simulink model "MR_SOC_SOP_SOE_Estimator"  (R2022b)
settings: Solver=VariableStepAuto  StartTime=0.0  StopTime=10.0  RelTol=1e-3
undefined symbols (not defined in the file): Initial_Covariance, L_SOP, MaxChargeCurrent, MaxDischargeCurrent, Measurement_Noise_Covariance, NumberSt, NumModules, NumParallel, NumSeries, OCV_25, Process_Noise_Covariance, SOC_Max, SOC_Min, SOC_Vec1, SOH_Vec, Temperature_Vec, Ts, Ts_SOP, Vmax, Vmin
settings Model: DataDictionary=Estimators_Dictionary.sldd  Creator=japerez  LastModifiedBy=jgavidia
settings DebuggingCC: ParameterPrecisionLossMsg=none

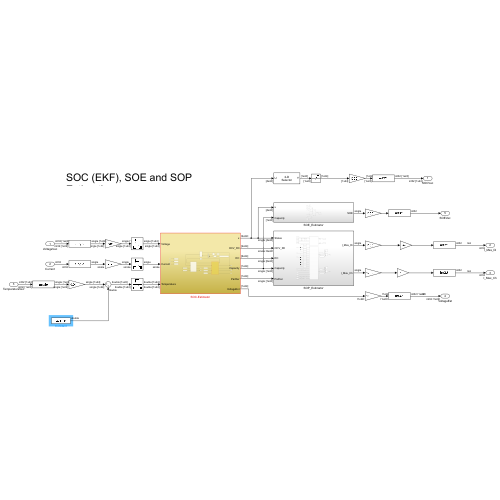
[thumbnail: Simulink's stored preview of the top-level diagram]
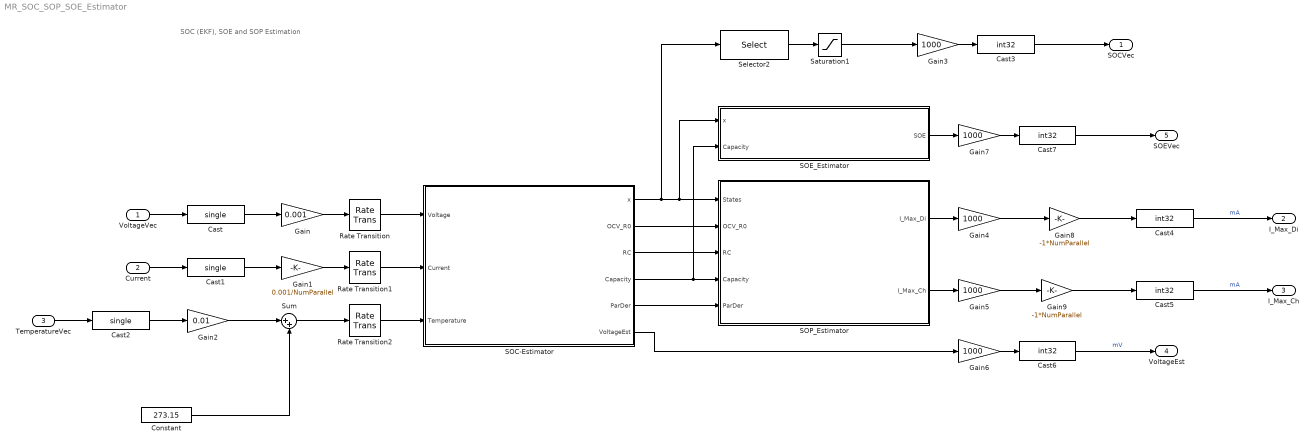
== system MR_SOC_SOP_SOE_Estimator ==
  note: SOC (EKF), SOE and SOP Estimation
  VoltageVec : Inport  OutDataTypeStr=int32  PortDimensions=[1,NumSeries*NumModules]
  Current : Inport  Port=2  OutDataTypeStr=int32  PortDimensions=1
  TemperatureVec : Inport  Port=3  OutDataTypeStr=int32  PortDimensions=[1,NumSeries*NumModules]
  Cast : DataTypeConversion  OutDataTypeStr=single  SaturateOnIntegerOverflow=off  RndMeth=Floor
  Cast1 : DataTypeConversion  OutDataTypeStr=single  SaturateOnIntegerOverflow=off  RndMeth=Floor
  Cast2 : DataTypeConversion  OutDataTypeStr=single  SaturateOnIntegerOverflow=off  RndMeth=Floor
  Cast{3..7} (5 alike) : DataTypeConversion  OutDataTypeStr=int32  SaturateOnIntegerOverflow=off  RndMeth=Floor
  Constant : Constant  Value=273.15  OutDataTypeStr=single
  Gain : Gain  Gain=0.001
  Gain1 : Gain  Gain=0.001/NumParallel
  Gain2 : Gain  Gain=0.01
  Gain{3..7} (5 alike) : Gain  Gain=1000
  Gain8 : Gain  Gain=-1*NumParallel
  Gain9 : Gain  Gain=-1*NumParallel
  Rate Transition : RateTransition  Integrity=off  OutPortSampleTime=Ts
  Rate Transition1 : RateTransition  Integrity=off  OutPortSampleTime=Ts
  Rate Transition2 : RateTransition  Integrity=off  OutPortSampleTime=Ts
  SOC-Estimator : Subsystem
  SOE_Estimator : Subsystem
  SOP_Estimator : Subsystem
  Saturation1 : Saturate  UpperLimit=1  LowerLimit=0
  Selector2 : Selector  NumberOfDimensions=2  InputPortWidth=24  IndexOptions=Index vector (dialog),Select all  Indices=1,1  OutputSizes=1,1
  Sum : Sum  Inputs=|++
  SOCVec : Outport  OutDataTypeStr=int32  PortDimensions=[1,NumSeries*NumModules]
  I_Max_Di : Outport  Port=2  OutDataTypeStr=int32  PortDimensions=1
  I_Max_Ch : Outport  Port=3  OutDataTypeStr=int32  PortDimensions=1
  VoltageEst : Outport  Port=4  OutDataTypeStr=int32  PortDimensions=[1,NumSeries*NumModules]
  SOEVec : Outport  Port=5
  wires:
  Gain/1 -> Rate Transition/1
  Rate Transition2/1 -> SOC-Estimator/3(Temperature)
  Gain1/1 -> Rate Transition1/1
  Selector2/1 -> Saturation1/1
  VoltageVec/1 -> Cast/1
  Current/1 -> Cast1/1
  TemperatureVec/1 -> Cast2/1
  Cast/1 -> Gain/1
  Cast1/1 -> Gain1/1
  Cast2/1 -> Gain2/1
  Gain3/1 -> Cast3/1
  Saturation1/1 -> Gain3/1
  SOC-Estimator/1(x) -> SOE_Estimator/1(x), SOP_Estimator/1(States), Selector2/1
  SOC-Estimator/2(OCV_R0) -> SOP_Estimator/2(OCV_R0)
  SOC-Estimator/3(RC) -> SOP_Estimator/3(RC)
  SOC-Estimator/4(Capacity) -> SOE_Estimator/2(Capacity), SOP_Estimator/4(Capacity)
  SOC-Estimator/5(ParDer) -> SOP_Estimator/5(ParDer)
  SOP_Estimator/1(I_Max_Di) -> Gain4/1
  SOP_Estimator/2(I_Max_Ch) -> Gain5/1
  Gain6/1 -> Cast6/1
  SOC-Estimator/6(VoltageEst) -> Gain6/1
  Rate Transition1/1 -> SOC-Estimator/2(Current)
  Rate Transition/1 -> SOC-Estimator/1(Voltage)
  Cast3/1 -> SOCVec/1
  Cast4/1 -> I_Max_Di/1  "mA"
  Cast5/1 -> I_Max_Ch/1  "mA"
  Cast6/1 -> VoltageEst/1  "mV"
  SOE_Estimator/1(SOE) -> Gain7/1
  Gain7/1 -> Cast7/1
  Cast7/1 -> SOEVec/1
  Constant/1 -> Sum/2
  Gain2/1 -> Sum/1
  Sum/1 -> Rate Transition2/1
  Gain5/1 -> Gain9/1
  Gain9/1 -> Cast5/1
  Gain4/1 -> Gain8/1
  Gain8/1 -> Cast4/1

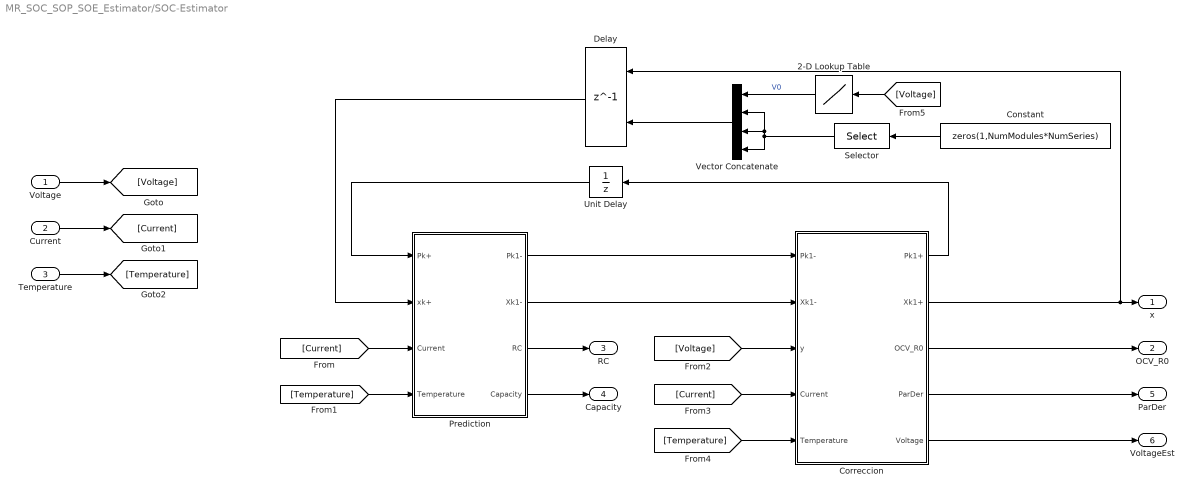
== system MR_SOC_SOP_SOE_Estimator/SOC-Estimator ==
  Voltage : Inport
  Current : Inport  Port=2
  Temperature : Inport  Port=3
  2-D Lookup Table : Lookup_n-D  NumberOfTableDimensions=1  BreakpointsForDimension1=OCV_25  BreakpointsForDimension2=Temperature_Vec  BreakpointsForDimension3=SOH_Vec  Table=SOC_Vec1  ExtrapMethod=Clip  InternalRulePriority=Speed  RndMeth=Simplest
  Constant : Constant  Value=zeros(1,NumModules*NumSeries)  OutDataTypeStr=single
  Correccion : Subsystem
  Delay : Delay  DelayLength=1  InitialConditionSource=Input port
      settings: InputPortMap=u0,p4
  Prediction : Subsystem
  Selector : Selector  NumberOfDimensions=2  InputPortWidth=3  IndexOptions=Select all,Index vector (dialog)  Indices=[1 3],[1:24]  OutputSizes=1,1
  Unit Delay : UnitDelay  InitialCondition=Initial_Covariance.*ones(NumberSt, NumModules*NumSeries)  SampleTime=Ts  HasFrameUpgradeWarning=on
  Vector Concatenate : Concatenate  NumInputs=4  Mode=Multidimensional array
  x : Outport
  OCV_R0 : Outport  Port=2
  RC : Outport  Port=3
  Capacity : Outport  Port=4
  ParDer : Outport  Port=5
  VoltageEst : Outport  Port=6
  wires:
  [Current] -> Prediction/3(Current)
  [Temperature] -> Prediction/4(Temperature)
  Temperature/1 -> [Temperature]
  Correccion/1(Pk1+) -> Unit Delay/1
  Prediction/1(Pk1-) -> Correccion/1(Pk1-)
  Prediction/2(Xk1-) -> Correccion/2(Xk1-)
  Correccion/2(Xk1+) -> Delay/1, x/1
  [Voltage] -> Correccion/3(y)
  Voltage/1 -> [Voltage]
  Current/1 -> [Current]
  Unit Delay/1 -> Prediction/1(Pk+)
  [Temperature] -> Correccion/5(Temperature)
  [Current] -> Correccion/4(Current)
  Correccion/3(OCV_R0) -> OCV_R0/1
  Delay/1 -> Prediction/2(xk+)
  Prediction/3(RC) -> RC/1
  Prediction/4(Capacity) -> Capacity/1
  Correccion/4(ParDer) -> ParDer/1
  Correccion/5(Voltage) -> VoltageEst/1
  Constant/1 -> Selector/1
  2-D Lookup Table/1 -> Vector Concatenate/1  "V0"
  Vector Concatenate/1 -> Delay/2
  [Voltage] -> 2-D Lookup Table/1
  Selector/1 -> Vector Concatenate/2, Vector Concatenate/3, Vector Concatenate/4

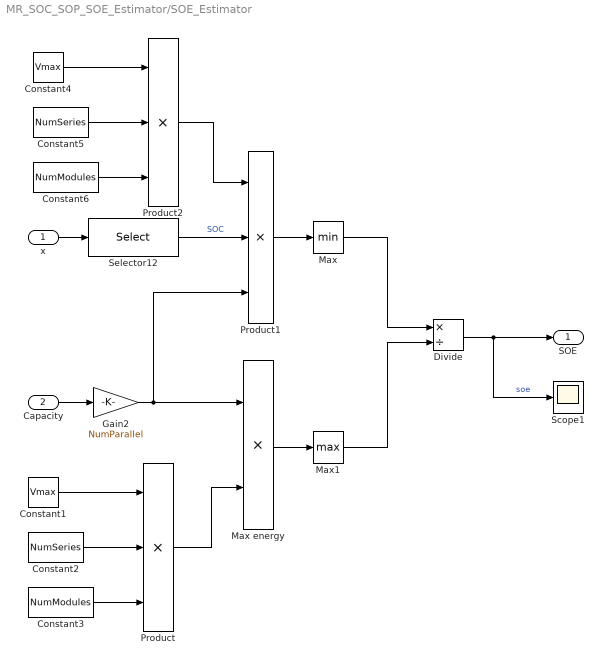
== system MR_SOC_SOP_SOE_Estimator/SOE_Estimator ==
  x : Inport
  Capacity : Inport  Port=2
  Constant1 : Constant  Value=Vmax
  Constant2 : Constant  Value=NumSeries
  Constant3 : Constant  Value=NumModules
  Constant4 : Constant  Value=Vmax
  Constant5 : Constant  Value=NumSeries
  Constant6 : Constant  Value=NumModules
  Divide : Product  Inputs=*/
  Gain2 : Gain  Gain=NumParallel
  Max : MinMax
  Max energy : Product
  Max1 : MinMax  Function=max
  Product : Product  Inputs=3
  Product1 : Product  Inputs=3
  Product2 : Product  Inputs=3
  Scope1 : Scope
  Selector12 : Selector  NumberOfDimensions=2  InputPortWidth=24  IndexOptions=Index vector (dialog),Select all  Indices=1,1  OutputSizes=1,1
  SOE : Outport  OutDataTypeStr=single
  wires:
  x/1 -> Selector12/1
  Constant1/1 -> Product/1
  Constant2/1 -> Product/2
  Capacity/1 -> Gain2/1
  Product/1 -> Max energy/2
  Max/1 -> Divide/1
  Max1/1 -> Divide/2
  Divide/1 -> SOE/1, Scope1/1  "soe"
  Product1/1 -> Max/1
  Max energy/1 -> Max1/1
  Constant3/1 -> Product/3
  Selector12/1 -> Product1/2  "SOC"
  Constant6/1 -> Product2/3
  Constant5/1 -> Product2/2
  Constant4/1 -> Product2/1
  Product2/1 -> Product1/1
  Gain2/1 -> Product1/3, Max energy/1

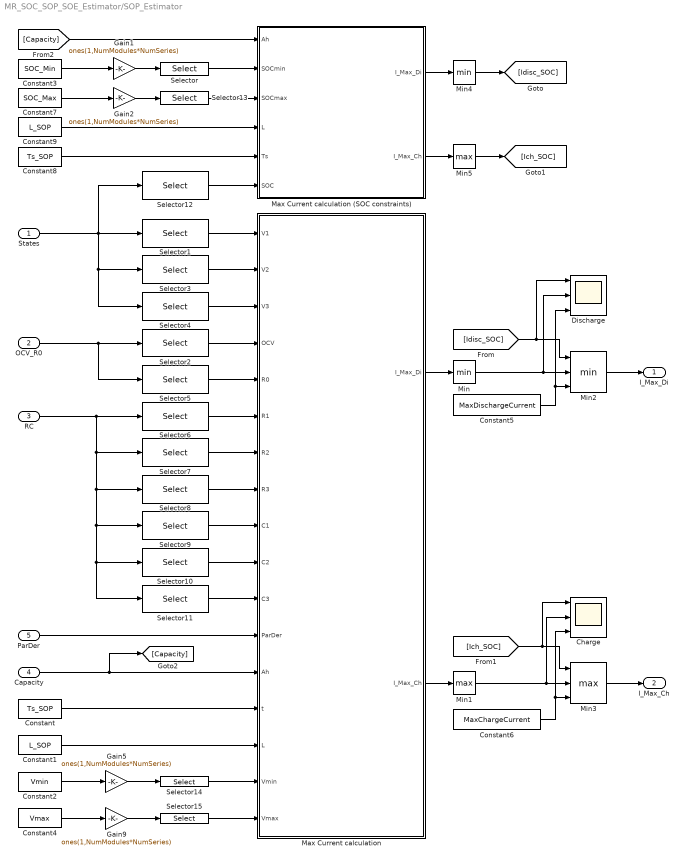
== system MR_SOC_SOP_SOE_Estimator/SOP_Estimator ==
  States : Inport  OutDataTypeStr=single  PortDimensions=[NumberSt, NumModules*NumSeries]
  OCV_R0 : Inport  Port=2  OutDataTypeStr=single  PortDimensions=[2,NumModules*NumSeries]
  RC : Inport  Port=3  OutDataTypeStr=single  PortDimensions=[6,NumModules*NumSeries]
  Capacity : Inport  Port=4  OutDataTypeStr=single  PortDimensions=[1,NumModules*NumSeries]
  ParDer : Inport  Port=5  OutDataTypeStr=single  PortDimensions=[1,NumModules*NumSeries]
  Charge : Scope  NumInputPorts=3
  Constant : Constant  Value=Ts_SOP
  Constant1 : Constant  Value=L_SOP
  Constant2 : Constant  Value=Vmin  OutDataTypeStr=single
  Constant3 : Constant  Value=SOC_Min  OutDataTypeStr=single
  Constant4 : Constant  Value=Vmax  OutDataTypeStr=single
  Constant5 : Constant  Value=MaxDischargeCurrent
  Constant6 : Constant  Value=MaxChargeCurrent
  Constant7 : Constant  Value=SOC_Max  OutDataTypeStr=single
  Constant8 : Constant  Value=Ts_SOP
  Constant9 : Constant  Value=L_SOP
  Discharge : Scope  NumInputPorts=3
  Gain{1..2,5,9} (4 alike) : Gain  Gain=ones(1,NumModules*NumSeries)  ParamDataTypeStr=single  OutDataTypeStr=single
  Max Current calculation : MATLAB Function  TreatAsAtomicUnit=on
  Max Current calculation (SOC constraints) : MATLAB Function  TreatAsAtomicUnit=on
  Min : MinMax
  Min1 : MinMax  Function=max
  Min2 : MinMax  Inputs=3
  Min3 : MinMax  Function=max  Inputs=3
  Min4 : MinMax
  Min5 : MinMax  Function=max
  Selector{,13..15} (4 alike) : Selector  NumberOfDimensions=2  InputPortWidth=3  IndexOptions=Index vector (dialog),Select all  Indices=1,1  OutputSizes=1,1
  Selector1 : Selector  NumberOfDimensions=2  InputPortWidth=24  IndexOptions=Index vector (dialog),Select all  Indices=2,2  OutputSizes=1,1
  Selector10 : Selector  NumberOfDimensions=2  InputPortWidth=24  IndexOptions=Index vector (dialog),Select all  Indices=5,5  OutputSizes=1,1
  Selector11 : Selector  NumberOfDimensions=2  InputPortWidth=24  IndexOptions=Index vector (dialog),Select all  Indices=6,6  OutputSizes=1,1
  Selector12 : Selector  NumberOfDimensions=2  InputPortWidth=24  IndexOptions=Index vector (dialog),Select all  Indices=1,1  OutputSizes=1,1
  Selector2 : Selector  NumberOfDimensions=2  InputPortWidth=24  IndexOptions=Index vector (dialog),Select all  Indices=1,1  OutputSizes=1,1
  Selector3 : Selector  NumberOfDimensions=2  InputPortWidth=24  IndexOptions=Index vector (dialog),Select all  Indices=3,3  OutputSizes=1,1
  Selector4 : Selector  NumberOfDimensions=2  InputPortWidth=24  IndexOptions=Index vector (dialog),Select all  Indices=4,4  OutputSizes=1,1
  Selector5 : Selector  NumberOfDimensions=2  InputPortWidth=24  IndexOptions=Index vector (dialog),Select all  Indices=2,2  OutputSizes=1,1
  Selector6 : Selector  NumberOfDimensions=2  InputPortWidth=24  IndexOptions=Index vector (dialog),Select all  Indices=1,1  OutputSizes=1,1
  Selector7 : Selector  NumberOfDimensions=2  InputPortWidth=24  IndexOptions=Index vector (dialog),Select all  Indices=2,2  OutputSizes=1,1
  Selector8 : Selector  NumberOfDimensions=2  InputPortWidth=24  IndexOptions=Index vector (dialog),Select all  Indices=3,3  OutputSizes=1,1
  Selector9 : Selector  NumberOfDimensions=2  InputPortWidth=24  IndexOptions=Index vector (dialog),Select all  Indices=4,4  OutputSizes=1,1
  I_Max_Di : Outport  OutDataTypeStr=single  PortDimensions=1
  I_Max_Ch : Outport  Port=2  OutDataTypeStr=single  PortDimensions=1
  wires:
  Selector1/1 -> Max Current calculation/1(V1)
  Selector5/1 -> Max Current calculation/5(R0)
  Constant2/1 -> Gain5/1
  Max Current calculation/2(I_Max_Ch) -> Min1/1
  Min2/1 -> I_Max_Di/1
  Max Current calculation/1(I_Max_Di) -> Min/1
  Constant4/1 -> Gain9/1
  OCV_R0/1 -> Selector5/1, Selector2/1
  Gain5/1 -> Selector14/1
  Capacity/1 -> [Capacity], Max Current calculation/13(Ah)
  Selector3/1 -> Max Current calculation/2(V2)
  Min3/1 -> I_Max_Ch/1
  RC/1 -> Selector11/1, Selector10/1, Selector9/1, Selector8/1, Selector7/1, Selector6/1
  Selector2/1 -> Max Current calculation/4(OCV)
  Selector6/1 -> Max Current calculation/6(R1)
  Selector11/1 -> Max Current calculation/11(C3)
  Selector10/1 -> Max Current calculation/10(C2)
  Selector9/1 -> Max Current calculation/9(C1)
  ParDer/1 -> Max Current calculation/12(ParDer)
  Selector8/1 -> Max Current calculation/8(R3)
  Selector7/1 -> Max Current calculation/7(R2)
  Selector4/1 -> Max Current calculation/3(V3)
  Constant1/1 -> Max Current calculation/15(L)
  Gain9/1 -> Selector15/1
  Constant3/1 -> Gain1/1
  States/1 -> Selector12/1, Selector4/1, Selector3/1, Selector1/1
  Constant7/1 -> Gain2/1
  Selector12/1 -> Max Current calculation (SOC constraints)/6(SOC)
  Gain2/1 -> Selector13/1
  Gain1/1 -> Selector/1
  Max Current calculation (SOC constraints)/1(I_Max_Di) -> Min4/1
  Max Current calculation (SOC constraints)/2(I_Max_Ch) -> Min5/1
  Min4/1 -> [Idisc_SOC]
  Min5/1 -> [Ich_SOC]
  Min/1 -> Discharge/2, Min2/2
  [Idisc_SOC] -> Discharge/1, Min2/1
  Constant6/1 -> Min3/3, Charge/3
  [Ich_SOC] -> Charge/1, Min3/1
  [Capacity] -> Max Current calculation (SOC constraints)/1(Ah)
  Min1/1 -> Charge/2, Min3/2
  Constant5/1 -> Discharge/3, Min2/3
  Constant9/1 -> Max Current calculation (SOC constraints)/4(L)
  Constant8/1 -> Max Current calculation (SOC constraints)/5(Ts)
  Constant/1 -> Max Current calculation/14(t)
  Selector/1 -> Max Current calculation (SOC constraints)/2(SOCmin)
  Selector13/1 -> Max Current calculation (SOC constraints)/3(SOCmax)
  Selector14/1 -> Max Current calculation/16(Vmin)
  Selector15/1 -> Max Current calculation/17(Vmax)

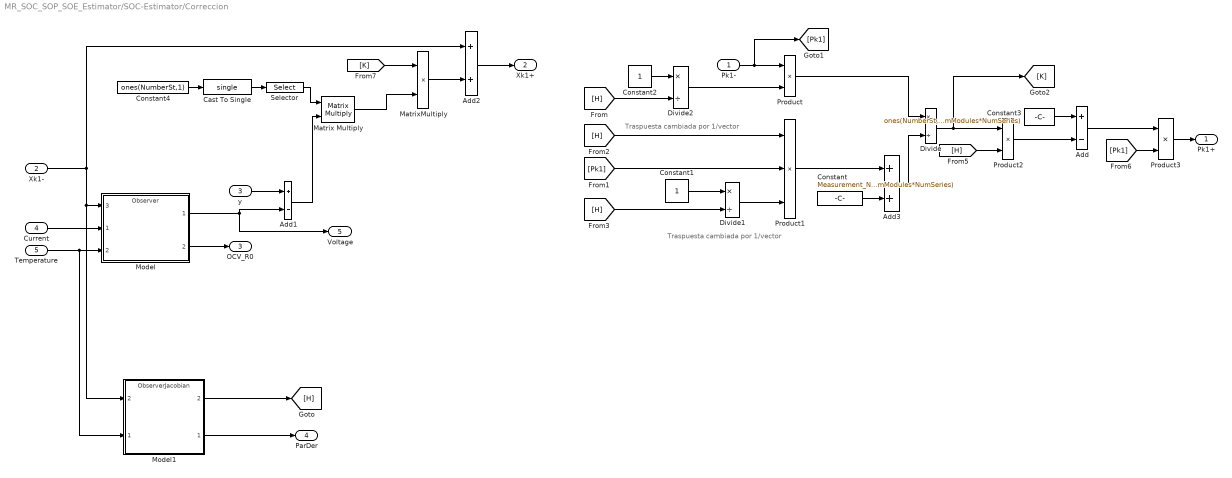
== system MR_SOC_SOP_SOE_Estimator/SOC-Estimator/Correccion ==
  note: Traspuesta cambiada por 1/vector
  note: Traspuesta cambiada por 1/vector
  Pk1- : Inport
  Xk1- : Inport  Port=2
  y : Inport  Port=3
  Current : Inport  Port=4
  Temperature : Inport  Port=5
  Add : Sum  Inputs=+-
  Add1 : Sum  Inputs=+-
  Add2 : Sum
  Add3 : Sum
  Cast To Single : DataTypeConversion  OutDataTypeStr=single  SaturateOnIntegerOverflow=off  RndMeth=Floor
  Constant : Constant  Value=Measurement_Noise_Covariance.*ones(1,NumModules*NumSeries)
  Constant1 : Constant  OutDataTypeStr=single
  Constant2 : Constant  OutDataTypeStr=single
  Constant3 : Constant  Value=ones(NumberSt,NumModules*NumSeries)  OutDataTypeStr=single
  Constant4 : Constant  Value=ones(NumberSt,1)
  Divide : Product  Inputs=*/
  Divide1 : Product  Inputs=*/
  Divide2 : Product  Inputs=*/
  Matrix Multiply : Product  Multiplication=Matrix(*)
  MatrixMultiply : Product
  Model : ModelReference  ModelNameDialog=Observer.slx  SimulationMode=Normal  ModelReferenceVersion=1.68
      settings: PortSchema="{\"entries\":[{\"content\":{\"sides\":[{\"content\":{\"connectorIds\":[\"In3\",\"In1\",\"In2\"]},\"type\":\"ConnectorPlacement.EquallySpacedRectSide\",\"uuid\":\"578ab670-1fda-43cf-957f-d385bd038916\"},{\"content\":{\"connectorIds\":[\"Out1\",\"Out2\"],\"side\":\"RIGHT\"},\"type\":\"ConnectorPlacement.EquallySpacedRectSide\",\"uuid\":\"4b969430-feda-42b7-9c79-ebef60756efb\"},{\"content\":{\"connectorIds\":[],\"side\":\"TOP\"},\"type\":\"ConnectorPlacement.EquallySpacedRectSide\",\"uuid\":\"4cac5d2b-0234-4ed0-b02b-747a59c7157b\"}]},\"type\":\"ConnectorPlacement.EquallySpacedConnector\",\"uuid\":\"85d93a1c-d19f-40da-bbe5-909812e617d2\"}],\"packageUris\":[\"http://schema.mathworks.com/mf0/Connector/R2020b\"],\"version\":\"1.0\"}"
  Model1 : ModelReference  ModelNameDialog=ObserverJacobian.slx  SimulationMode=Normal  ModelReferenceVersion=1.67
      settings: PortSchema="{\"entries\":[{\"content\":{\"sides\":[{\"content\":{\"connectorIds\":[\"In2\",\"In1\"]},\"type\":\"ConnectorPlacement.EquallySpacedRectSide\",\"uuid\":\"624b1806-31b3-4d4e-aaed-5849830d0be2\"},{\"content\":{\"connectorIds\":[\"Out2\",\"Out1\"],\"side\":\"RIGHT\"},\"type\":\"ConnectorPlacement.EquallySpacedRectSide\",\"uuid\":\"bbfd7499-df97-4924-a8a8-c1065b8018b2\"},{\"content\":{\"connectorIds\":[],\"side\":\"TOP\"},\"type\":\"ConnectorPlacement.EquallySpacedRectSide\",\"uuid\":\"a9ee114e-551d-4138-9f4b-27e93fc3876b\"}]},\"type\":\"ConnectorPlacement.EquallySpacedConnector\",\"uuid\":\"be93e1de-0c8b-49c5-8782-6d924248437e\"}],\"packageUris\":[\"http://schema.mathworks.com/mf0/Connector/R2020b\"],\"version\":\"1.0\"}"
  Product : Product
  Product1 : Product  Inputs=3
  Product2 : Product
  Product3 : Product
  Selector : Selector  NumberOfDimensions=2  InputPortWidth=3  IndexOptions=Index vector (dialog),Select all  Indices=[1 2 3 4],1  OutputSizes=1,1
  Pk1+ : Outport
  Xk1+ : Outport  Port=2
  OCV_R0 : Outport  Port=3
  ParDer : Outport  Port=4
  Voltage : Outport  Port=5
  wires:
  Pk1-/1 -> [Pk1], Product/1
  Model1/2 -> [H]
  Divide2/1 -> Product/2
  Product/1 -> Divide/1
  [H] -> Product1/1
  [Pk1] -> Product1/2
  Divide1/1 -> Product1/3
  Product1/1 -> Add3/1
  Product2/1 -> Add/2
  [H] -> Product2/2
  Add/1 -> Product3/1
  [Pk1] -> Product3/2
  Product3/1 -> Pk1+/1
  y/1 -> Add1/1
  Model/1 -> Add1/2, Voltage/1
  MatrixMultiply/1 -> Add2/2
  Xk1-/1 -> Model1/2, Model/3, Add2/1
  Add2/1 -> Xk1+/1
  Add3/1 -> Divide/2
  Current/1 -> Model/1
  Temperature/1 -> Model1/1, Model/2
  Constant1/1 -> Divide1/1
  [H] -> Divide1/2
  [H] -> Divide2/2
  Constant2/1 -> Divide2/1
  Constant3/1 -> Add/1
  [K] -> MatrixMultiply/1
  Model/2 -> OCV_R0/1
  Model1/1 -> ParDer/1
  Divide/1 -> [K], Product2/1
  Constant/1 -> Add3/2
  Matrix Multiply/1 -> MatrixMultiply/2
  Add1/1 -> Matrix Multiply/2
  Constant4/1 -> Cast To Single/1
  Cast To Single/1 -> Selector/1
  Selector/1 -> Matrix Multiply/1

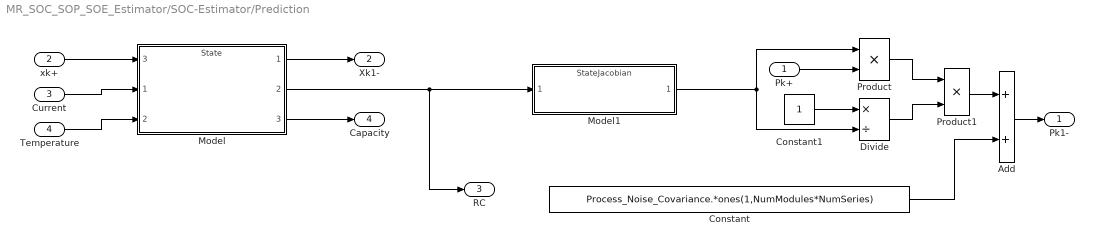
== system MR_SOC_SOP_SOE_Estimator/SOC-Estimator/Prediction ==
  Pk+ : Inport
  xk+ : Inport  Port=2
  Current : Inport  Port=3
  Temperature : Inport  Port=4
  Add : Sum
  Constant : Constant  Value=Process_Noise_Covariance.*ones(1,NumModules*NumSeries)
  Constant1 : Constant  OutDataTypeStr=single
  Divide : Product  Inputs=*/
  Model : ModelReference  ModelNameDialog=State.slx  SimulationMode=Normal  ModelReferenceVersion=1.71
      settings: PortSchema="{\"entries\":[{\"content\":{\"sides\":[{\"content\":{\"connectorIds\":[\"In3\",\"In1\",\"In2\"]},\"type\":\"ConnectorPlacement.EquallySpacedRectSide\",\"uuid\":\"c0b7b42f-4c9c-4d33-8f89-0d8f101f18a4\"},{\"content\":{\"connectorIds\":[\"Out1\",\"Out2\",\"Out3\"],\"side\":\"RIGHT\"},\"type\":\"ConnectorPlacement.EquallySpacedRectSide\",\"uuid\":\"5a15646a-ccfe-4412-8f35-1662de2d0b3b\"},{\"content\":{\"connectorIds\":[],\"side\":\"TOP\"},\"type\":\"ConnectorPlacement.EquallySpacedRectSide\",\"uuid\":\"17dc4d1a-17c1-45d9-9053-5b2c4d4501d0\"}]},\"type\":\"ConnectorPlacement.EquallySpacedConnector\",\"uuid\":\"a8287c94-104f-4768-a086-94df798e70cd\"}],\"packageUris\":[\"http://schema.mathworks.com/mf0/Connector/R2020b\"],\"version\":\"1.0\"}"
  Model1 : ModelReference  ModelNameDialog=StateJacobian.slx  SimulationMode=Normal  ModelReferenceVersion=1.69
  Product : Product
  Product1 : Product
  Pk1- : Outport
  Xk1- : Outport  Port=2
  RC : Outport  Port=3
  Capacity : Outport  Port=4
  wires:
  Pk+/1 -> Product/2
  xk+/1 -> Model/3
  Temperature/1 -> Model/2
  Current/1 -> Model/1
  Model1/1 -> Divide/2, Product/1
  Divide/1 -> Product1/2
  Product/1 -> Product1/1
  Product1/1 -> Add/1
  Model/1 -> Xk1-/1
  Add/1 -> Pk1-/1
  Constant1/1 -> Divide/1
  Model/2 -> Model1/1, RC/1
  Model/3 -> Capacity/1
  Constant/1 -> Add/2

== matlab function MR_SOC_SOP_SOE_Estimator/SOP_Estimator/Max Current calculation ==
  data: V1 input; V2 input; V3 input; OCV input single; R0 input single; R1 input single; R2 input single; R3 input single; C1 input single; C2 input single; C3 input single; ParDer input; Ah input single; I_Max_Di output single; t input; L input; Vmin input; Vmax input; I_Max_Ch output single
function [I_Max_Di,I_Max_Ch] = fcn(V1,V2,V3,OCV,R0,R1,R2,R3,C1,C2,C3,ParDer,Ah,t,L,Vmin,Vmax)

% Temporal constants
tau1=R1.*C1;
tau2=R2.*C2;
tau3=R3.*C3;
% Equations
Numerator= OCV-V1.*exp((-L*t)./tau1)-V2.*exp((-L*t)./tau2)-V3.*exp((-L*t)./tau3);
Denominator= ((L*t./(Ah*3600)).*ParDer)+R0+R1.*(1-exp((-L*t)./tau1))+R2.*(1-exp((-L*t)./tau2))+R3.*(1-exp((-L*t)./tau3));

I_Max_Di = (Numerator-Vmin)./Denominator;

I_Max_Ch = (Numerator-Vmax)./Denominator;

== matlab function MR_SOC_SOP_SOE_Estimator/SOP_Estimator/Max Current calculation (SOC constraints) ==
  data: Ah input; I_Max_Di output; SOCmin input; SOCmax input; L input; Ts input; I_Max_Ch output; SOC input
function [I_Max_Di, I_Max_Ch]= fcn(Ah,SOCmin,SOCmax,L,Ts,SOC)

Numerator_dis= SOC-SOCmin;
Numerator_ch= SOC-SOCmax;
Denominator= (L*Ts)./(Ah*3600);

I_Max_Di = Numerator_dis./Denominator;

I_Max_Ch = Numerator_ch./Denominator;
